simulink model "rectifier_design"  (R2025a)
settings: Solver=VariableStepAuto  StartTime=0.0  StopTime=0.2  RelTol=1e-3
libraries: spsDiodeLib x4, spsSeriesRLCBranchLib x3, spsCurrentMeasurementLib x2, spsACVoltageSourceLib x1, spsGroundLib x1, spsMeanLib x1, spsVoltageMeasurementLib x1, sps_lib x1
settings Model: Creator=Lenovo  LastModifiedBy=Lenovo

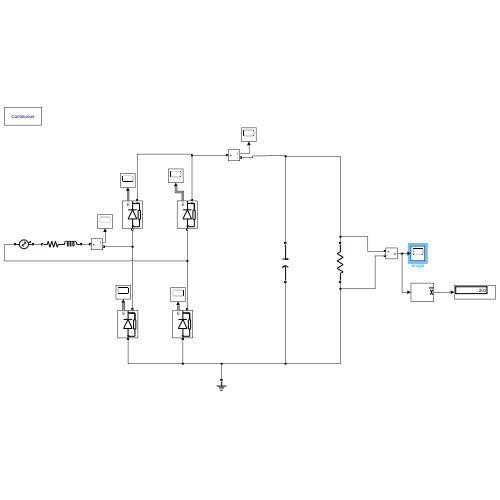
[thumbnail: Simulink's stored preview of the top-level diagram]
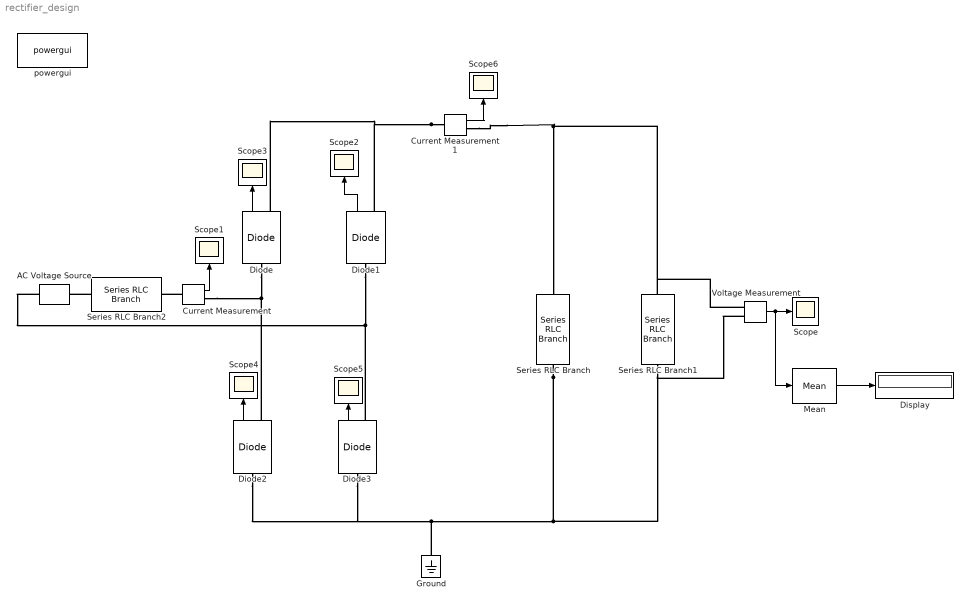
== system rectifier_design ==
  AC Voltage Source : spsACVoltageSourceLib/AC Voltage Source  Amplitude=215  Phase=0  Frequency=50  SampleTime=0  Measurements=None  BusType=swing  Pref=10e3  Qref=0  Qmin=-inf  Qmax=+inf
  Current Measurement : spsCurrentMeasurementLib/Current Measurement  PhasorSimulation=off  OutputType=Complex  PSBequivalent=0
  Current Measurement1 : spsCurrentMeasurementLib/Current Measurement  PhasorSimulation=off  OutputType=Complex  PSBequivalent=0
  Diode{,1..3} (4 alike) : spsDiodeLib/Diode  Ron=0.036  Lon=0  Vf=1.1  IC=0  UseSnubber=0  Rs=500  Cs=250e-9  Measurements=on
  Display : Display
  Ground : spsGroundLib/Ground  LConnTagsString=a
  Mean : spsMeanLib/Mean  Freq=60  Vinit=0  Ts=0
  Scope{,1..6} (7 alike) : Scope
      Scope settings: ActiveDisplayYMinimum=-37.504825428405944  ActiveDisplayYMaximum=337.54342885565359
      Scope1 settings: ActiveDisplayYMinimum=-40.6124656236994  ActiveDisplayYMaximum=164.29455570774294
      Scope2 settings: ActiveDisplayYMinimum=-236.61883350471254  ActiveDisplayYMaximum=126.52753162504482  DataLoggingVariableName=ScopeData2
      Scope3 settings: ActiveDisplayYMinimum=-287.00698047954393  ActiveDisplayYMaximum=191.64559463687868  DataLoggingVariableName=ScopeData3
      Scope4 settings: ActiveDisplayYMinimum=-236.61883350471254  ActiveDisplayYMaximum=126.52753162504482  DataLoggingVariableName=ScopeData4
      Scope5 settings: ActiveDisplayYMinimum=-317.56132708157151  ActiveDisplayYMaximum=847.43866821622464  DataLoggingVariableName=ScopeData5
      Scope6 settings: ActiveDisplayYMinimum=-17.970873212055253  ActiveDisplayYMaximum=161.72667079451179  DataLoggingVariableName=ScopeData6
  Series RLC Branch : spsSeriesRLCBranchLib/Series RLC Branch  LConnTagsString=__new0  RConnTagsString=__new0  BranchType=C  Resistance=1  Inductance=1e-3  SetiL0=off  InitialCurrent=0  Capacitance=1500e-6  Setx0=off  InitialVoltage=0  Measurements=None
  Series RLC Branch1 : spsSeriesRLCBranchLib/Series RLC Branch  LConnTagsString=__new0  RConnTagsString=__new0  BranchType=R  Resistance=60  Inductance=1e-3  SetiL0=off  InitialCurrent=0  Capacitance=150e-6  Setx0=off  InitialVoltage=0  Measurements=None
  Series RLC Branch2 : spsSeriesRLCBranchLib/Series RLC Branch  LConnTagsString=__new0  RConnTagsString=__new0  BranchType=RL  Resistance=0.1  Inductance=1e-3  SetiL0=off  InitialCurrent=0  Capacitance=1e-6  Setx0=off  InitialVoltage=0  Measurements=None
  Voltage Measurement : spsVoltageMeasurementLib/Voltage Measurement  PhasorSimulation=off  OutputType=Complex  PSBequivalent=0
  powergui : sps_lib/powergui  Priority=1  SimulationMode=Continuous  SampleTime=50e-6  frequency=60  Iterations=50  frequencyindice=50  Pbase=100e6  ErrMax=1e-4  UnitsV=kV  UnitsW=MW  buscounter=0  FunctionMessages=off  echomessages=off  EnableUseOfTLC=off  CurrentSourceSwitches=off  DisableSnubberDevices=off  DisableRonSwitches=off  DisableVfSwitches=off  DisplayEquations=off  AutomaticDiscreteSolvers=off  SolverType=Tustin/Backward Euler (TBE)  Interpol=off  ExternalGateDelay=off  methode=off  Ts=100  x0status=blocks  SPID=on  SwTol=0  HookPort=off  NonlinearTolerance=1e-4  nMaxIteration=100  ContinueOnMaxIteration=off  RestoreLinks=warning  ResistiveCurrentMeasurement=off  Frange=[0:2:500]  Ylog=off  Xlog=on  ShowGrid=off  save=off  variable=ZData  structure=0  ZoomFFT=off  StartTime=0.0  cycles=1  DisplayStyle=1  fundamental=60  FreqAxis=off  MaxFrequency=1000  frequencyindicesteady=1  RmsSteady=1  display=off
  wires:
  Current Measurement/1 -> Scope1/1
  Voltage Measurement/1 -> Mean/1, Scope/1
  Mean/1 -> Display/1
  Diode1/1 -> Scope2/1
  Diode/1 -> Scope3/1
  Diode2/1 -> Scope4/1
  Diode3/1 -> Scope5/1
  Current Measurement1/1 -> Scope6/1
  connections:
  Voltage Measurement/LConn1 -- Series RLC Branch1/LConn1 -- Current Measurement1/RConn1 -- Series RLC Branch/LConn1
  Series RLC Branch/RConn1 -- Ground/LConn1 -- Diode3/LConn1 -- Diode2/LConn1 -- Voltage Measurement/LConn2 -- Series RLC Branch1/RConn1
  AC Voltage Source/LConn1 -- Diode3/RConn1 -- Diode1/LConn1
  Current Measurement/RConn1 -- Diode/LConn1 -- Diode2/RConn1
  Current Measurement1/LConn1 -- Diode1/RConn1 -- Diode/RConn1
  Current Measurement/LConn1 -- Series RLC Branch2/RConn1
  Series RLC Branch2/LConn1 -- AC Voltage Source/RConn1
